simulink model "filtro_ativo"  (R2017a)
settings: Solver=ode3  StartTime=0.0  StopTime=2  MaxStep=Ts  RelTol=1e-3
InitFcn:
  | Ts=1/60/3240;
libraries: powerlib x51, powerlib_meascontrol x3, dsparch4 x2, simulink x1
settings Model: ExtModeTrigMode=oneshot  ExtModeArmWhenConnect=off  ExtModeAutoUpdateStatusClock=off  Creator=patrice  LastModifiedBy=Familia
settings DataIOCC: SaveFormat=Array  SignalLoggingName=sigsOut
settings OptimizationCC: BlockReduction=off  BooleanDataType=off  ExpressionDepthLimit=2147483647  InitFltsAndDblsToZero=on  LifeSpan=inf
settings DebuggingCC: SaveWithParameterizedLinksMsg=none  UnderspecifiedInitializationDetection=Classic  MergeDetectMultiDrivingBlocksExec=none  CheckExecutionContextPreStartOutputMsg=on  CheckExecutionContextRuntimeOutputMsg=on  SignalResolutionControl=TryResolveAllWithWarning  MultiTaskDSMMsg=warning  MultiTaskCondExecSysMsg=none  FcnCallInpInsideContextMsg=warning  StateNameClashWarn=warning  SFUnexpectedBacktrackingDiag=warning  SFNoUnconditionalDefaultTransitionDiag=warning  SFExecutionAtInitializationDiag=none
settings HardwareCC: ProdBitPerPointer=32  ProdBitPerSizeT=32  ProdBitPerPtrDiffT=32  ProdLargestAtomicFloat=None  ProdIntDivRoundTo=Undefined  ProdEndianess=Unspecified  ProdWordSize=32  ProdHWDeviceType=32-bit Generic  TargetUnknown=on
settings ModelReferenceCC: PropagateSignalLabelsOutOfModel=off
settings GRTTargetCC: TargetFcnLib=ansi_tfl_tmw.mat  TargetLangStandard=C89/C90 (ANSI)  GeneratePreprocessorConditionals=Disable all  CombineOutputUpdateFcns=off  GRTInterface=on
settings ConfigComp: CovMetricSettings=dw  CovHtmlReporting=on  CovSaveCumulativeToWorkspaceVar=on  CovSaveSingleToWorkspaceVar=on  CovExternalEMLEnable=off

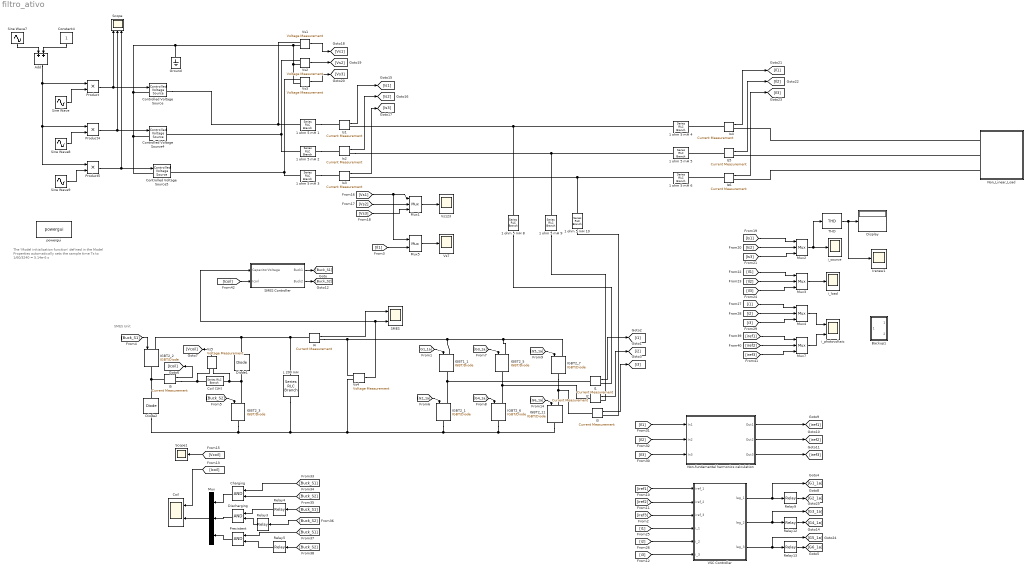
== system filtro_ativo ==
  note: SMES Unit
  note: The 'Model  initialization function' defined in the
      | Model Properties automatically sets the sample time Ts
      | to 1/60/3240 = 5.14e-6 s
  1 ohm 5 mH {1..6} (6 alike) : powerlib/Elements/Series RLC Branch  LConnTagsString=__new0  RConnTagsString=__new0  BranchType=RL  Resistance=0.1  Inductance=0.5e-03  SetiL0=off  InitialCurrent=0  Capacitance=[]  Setx0=off  InitialVoltage=0  Measurements=None
  1 ohm 5 mH 10 : powerlib/Elements/Series RLC Branch  LConnTagsString=__new0  RConnTagsString=__new0  BranchType=RL  Resistance=0.1  Inductance=5e-03  SetiL0=off  InitialCurrent=0  Capacitance=[]  Setx0=off  InitialVoltage=0  Measurements=None
  1 ohm 5 mH 8 : powerlib/Elements/Series RLC Branch  LConnTagsString=__new0  RConnTagsString=__new0  BranchType=RL  Resistance=0.1  Inductance=5e-03  SetiL0=off  InitialCurrent=0  Capacitance=[]  Setx0=off  InitialVoltage=0  Measurements=None
  1 ohm 5 mH 9 : powerlib/Elements/Series RLC Branch  LConnTagsString=__new0  RConnTagsString=__new0  BranchType=RL  Resistance=0.1  Inductance=5e-03  SetiL0=off  InitialCurrent=0  Capacitance=[]  Setx0=off  InitialVoltage=0  Measurements=None
  Add : Sum
  Backup1 : Subsystem
  Charging : Logic  AllPortsSameDT=off
  Coil : Scope  NumInputPorts=2
  "Coil (1H) " : powerlib/Elements/Series RLC Branch  LConnTagsString=__new0  RConnTagsString=__new0  BranchType=L  Resistance=0.1  Inductance=1  SetiL0=on  InitialCurrent=13.2  Capacitance=[]  Setx0=off  InitialVoltage=0  Measurements=None
  Constant4 : Constant
  Controlled Voltage Source : powerlib/Electrical Sources/Controlled Voltage Source  Initialize=on  Source_Type=AC  Amplitude=0  Phase=0  Frequency=0  Measurements=None
  Controlled Voltage Source4 : powerlib/Electrical Sources/Controlled Voltage Source  Initialize=on  Source_Type=AC  Amplitude=0  Phase=0  Frequency=0  Measurements=None
  Controlled Voltage Source5 : powerlib/Electrical Sources/Controlled Voltage Source  Initialize=on  Source_Type=AC  Amplitude=0  Phase=0  Frequency=0  Measurements=None
  Diode1 : powerlib/Power Electronics/Diode  Ron=1e-2  Lon=0  Vf=0.8  IC=0  UseSnubber=off  Rs=inf  Cs=0  Measurements=off
  Diode2 : powerlib/Power Electronics/Diode  Ron=1e-2  Lon=0  Vf=0.8  IC=0  UseSnubber=off  Rs=inf  Cs=0  Measurements=off
  Discharging : Logic  AllPortsSameDT=off
  Display : Display
  Ground : powerlib/Elements/Ground  LConnTagsString=a
  I{1..5} (5 alike) : powerlib/Measurements/Current Measurement  Tag=PoWeRsYsTeMmEaSuReMeNt  PhasorSimulation=off  OutputType=Magnitude  PSBequivalent=0
  IGBT1_1 : powerlib/Power Electronics/IGBT//Diode  Ron=1e-3  Rs=1e5  Cs=inf  Measurements=off
  IGBT2_{1..3,5..7,11} (7 alike) : powerlib/Power Electronics/IGBT//Diode  Ron=1e-3  Rs=1e5  Cs=inf  Measurements=off
  Irenew1 : Scope
  Is{1..6} (6 alike) : powerlib/Measurements/Current Measurement  Tag=PoWeRsYsTeMmEaSuReMeNt  PhasorSimulation=off  OutputType=Magnitude  PSBequivalent=0
  L 200 mH : powerlib/Elements/Series RLC Branch  LConnTagsString=__new0  RConnTagsString=__new0  BranchType=C  Resistance=1.0  Inductance=200e-03  SetiL0=off  InitialCurrent=0  Capacitance=1000e-9  Setx0=on  InitialVoltage=2000  Measurements=None
  Mux{,1..4,7} (6 alike) : Mux  Inputs=3
  Mux5 : Mux  Inputs=2
  Non-fundamental harmonics calculation : Subsystem
  Non_Linear_Load : Subsystem
  Precistent : Logic  AllPortsSameDT=off
  Product : Product
  Product4 : Product
  Product5 : Product
  Relay{3..5,9,12..13} (6 alike) : Relay  OnSwitchValue=0.5  OffSwitchValue=0.5  OnOutputValue=0  OffOutputValue=1
  "SMES " : Scope  NumInputPorts=2
  SMES Controller : Subsystem
  Scope : Scope  NumInputPorts=3
  Scope1 : Scope
  Sine Wave : Sin  Amplitude=230*sqrt(2)  Frequency=100*pi  SampleTime=0
  Sine Wave7 : Sin  Amplitude=0.3  Frequency=2*pi*5  SampleTime=0
  Sine Wave8 : Sin  Amplitude=230*sqrt(2)  Frequency=100*pi  Phase=-2*pi/3  SampleTime=0
  Sine Wave9 : Sin  Amplitude=230*sqrt(2)  Frequency=100*pi  Phase=2*pi/3  SampleTime=0
  THD : powerlib_meascontrol/Measurements/THD  Freq=50  Ts=0
  VSC Controller : Subsystem
  Vs{1..5} (5 alike) : powerlib/Measurements/Voltage Measurement  Tag=PoWeRsYsTeMmEaSuReMeNt  PhasorSimulation=off  OutputType=Magnitude  PSBequivalent=0
  Vs123 : Scope
  Vs7 : Scope
  i_load : Scope
  i_photovoltaic : Scope  NumInputPorts=2
  i_source : Scope
  powergui : powerlib/powergui  SimulationMode=Discrete  SampleTime=Ts  frequency=60  Iterations=50  frequencyindice=0  Pbase=100e6  ErrMax=1e-4  UnitsV=kV  UnitsW=MW  buscounter=0  FunctionMessages=off  echomessages=off  EnableUseOfTLC=off  CurrentSourceSwitches=off  DisableSnubberDevices=off  DisableRonSwitches=off  DisableVfSwitches=off  DisplayEquations=off  SolverType=Tustin  Interpol=off  ExternalGateDelay=off  methode=off  Ts=0  x0status=blocks  SPID=off  SwTol=0  HookPort=off  RestoreLinks=warning  ResistiveCurrentMeasurement=off  Frange=[0:2:500]  Ylog=off  Xlog=on  ShowGrid=off  save=off  variable=ZData  structure=sps1phPWM2_str  ZoomFFT=off  StartTime=0.2  cycles=2  DisplayStyle=2  fundamental=50  FreqAxis=off  MaxFrequency=5000  frequencyindicesteady=1  RmsSteady=1  display=off
  wires:
  [G1_1a] -> IGBT1_1/1
  [G2_1a] -> IGBT2_1/1
  [G3_1a] -> IGBT2_5/1
  [G4_1a] -> IGBT2_6/1
  [G5_1a] -> IGBT2_7/1
  [G6_1a] -> IGBT2_11/1
  I1/1 -> [i1]
  I2/1 -> [i2]
  I3/1 -> [i3]
  Mux1/1 -> Vs123/1
  Is1/1 -> [Is1]
  Is2/1 -> [Is2]
  Is3/1 -> [Is3]
  Vs2/1 -> [Vs2]
  Vs1/1 -> [Vs1]
  Vs3/1 -> [Vs3]
  [Vs1] -> Mux5/1, Mux1/1
  [Vs2] -> Mux1/2
  [Vs3] -> Mux1/3
  Is4/1 -> [Il1]
  Is5/1 -> [Il2]
  Is6/1 -> [Il3]
  [Il1] -> Mux5/2
  Mux5/1 -> Vs7/1
  Mux2/1 -> THD/1, i_source/1
  [Is1] -> Mux2/1
  [Is2] -> Mux2/2
  [Is3] -> Mux2/3
  Mux3/1 -> i_load/1
  [Il2] -> Mux3/2
  [Il3] -> Mux3/3
  Mux4/1 -> i_photovoltaic/1
  [i2] -> Mux4/2
  [i3] -> Mux4/3
  [Il1] -> Mux3/1
  Relay9/1 -> [G2_1a]
  Relay12/1 -> [G4_1a]
  Relay13/1 -> [G6_1a]
  VSC Controller/3(leg_3) -> [G5_1a], Relay13/1
  VSC Controller/1(leg_1) -> Relay9/1, [G1_1a]
  [iref1] -> VSC Controller/1(iref_1)
  [iref3] -> VSC Controller/3(iref_3)
  VSC Controller/2(leg_2) -> Relay12/1, [G3_1a]
  [iref2] -> VSC Controller/2(iref_2)
  [i1] -> VSC Controller/4(i_1)
  [i2] -> VSC Controller/5(i_2)
  [i3] -> VSC Controller/6(i_3)
  THD/1 -> Irenew1/1, Display/1
  Vs4/1 -> "SMES "/2, SMES Controller/1(CapacitorVoltage)
  [i1] -> Mux4/1
  Vs5/1 -> [Vcoil]
  [Buck_S2] -> IGBT2_3/1
  [Buck_S1] -> IGBT2_2/1
  I5/1 -> [Icoil]
  [Icoil] -> Coil/1
  I4/1 -> "SMES "/1
  [Buck_S1] -> Charging/1
  [Buck_S2] -> Charging/2
  [Buck_S1] -> Relay4/1
  [Buck_S2] -> Relay3/1
  Relay4/1 -> Discharging/1
  Relay3/1 -> Discharging/2
  [Buck_S2] -> Relay5/1
  Relay5/1 -> Precistent/2
  [Buck_S1] -> Precistent/1
  Charging/1 -> Mux/1
  Discharging/1 -> Mux/2
  Precistent/1 -> Mux/3
  Mux7/1 -> i_photovoltaic/2
  [iref1] -> Mux7/1
  [iref2] -> Mux7/2
  [iref3] -> Mux7/3
  [Il1] -> Non-fundamental harmonics calculation/1(In1)
  [Il2] -> Non-fundamental harmonics calculation/2(In2)
  [Il3] -> Non-fundamental harmonics calculation/3(In3)
  Non-fundamental harmonics calculation/1(Out1) -> [iref1]
  Non-fundamental harmonics calculation/2(Out2) -> [iref2]
  Non-fundamental harmonics calculation/3(Out3) -> [iref3]
  Constant4/1 -> Add/2
  Sine Wave7/1 -> Add/1
  Sine Wave8/1 -> Product4/2
  Product5/1 -> Controlled Voltage Source5/1, Scope/3
  Sine Wave9/1 -> Product5/2
  Sine Wave/1 -> Product/2
  Product4/1 -> Controlled Voltage Source4/1, Scope/2
  Product/1 -> Controlled Voltage Source/1, Scope/1
  Add/1 -> Product5/1, Product4/1, Product/1
  SMES Controller/1(Buck1) -> [Buck_S1]
  SMES Controller/2(Buck2) -> [Buck_S2]
  [Icoil] -> SMES Controller/2(Icoil)
  [Vcoil] -> Scope1/1
  Mux/1 -> Coil/2
  connections:
  I4/RConn1 -- IGBT1_1/LConn1 -- IGBT2_5/LConn1 -- IGBT2_7/LConn1 -- Vs4/LConn1
  IGBT2_6/LConn1 -- IGBT2_5/RConn1 -- I2/LConn1
  IGBT2_7/RConn1 -- IGBT2_11/LConn1 -- I3/LConn1
  I1/LConn1 -- IGBT1_1/RConn1 -- IGBT2_1/LConn1
  Vs1/LConn1 -- Controlled Voltage Source/RConn1 -- 1 ohm 5 mH 1/LConn1
  1 ohm 5 mH 1/RConn1 -- Is1/LConn1
  1 ohm 5 mH 3/RConn1 -- Is3/LConn1
  1 ohm 5 mH 2/RConn1 -- Is2/LConn1
  1 ohm 5 mH 8/RConn1 -- 1 ohm 5 mH 4/RConn1 -- Is1/RConn1
  Is5/LConn1 -- 1 ohm 5 mH 5/LConn1
  1 ohm 5 mH 6/RConn1 -- Is3/RConn1 -- 1 ohm 5 mH 10/RConn1
  1 ohm 5 mH 8/LConn1 -- I1/RConn1
  1 ohm 5 mH 9/LConn1 -- I2/RConn1
  1 ohm 5 mH 10/LConn1 -- I3/RConn1
  Non_Linear_Load/LConn1 -- Is4/RConn1
  Non_Linear_Load/LConn2 -- Is5/RConn1
  Non_Linear_Load/LConn3 -- Is6/RConn1
  Is4/LConn1 -- 1 ohm 5 mH 4/LConn1
  1 ohm 5 mH 5/RConn1 -- Is2/RConn1 -- 1 ohm 5 mH 9/RConn1
  Is6/LConn1 -- 1 ohm 5 mH 6/LConn1
  I5/LConn1 -- Diode2/RConn1 -- IGBT2_2/RConn1
  IGBT2_3/LConn1 -- Vs5/LConn2 -- "Coil (1H) "/RConn1 -- Diode1/LConn1
  I5/RConn1 -- Vs5/LConn1 -- "Coil (1H) "/LConn1
  L 200 mH/LConn1 -- I4/LConn1 -- Diode1/RConn1 -- IGBT2_2/LConn1
  L 200 mH/RConn1 -- Diode2/LConn1 -- IGBT2_3/RConn1 -- Vs4/LConn2 -- IGBT2_1/RConn1 -- IGBT2_6/RConn1 -- IGBT2_11/RConn1
  Vs2/LConn1 -- 1 ohm 5 mH 2/LConn1 -- Controlled Voltage Source4/RConn1
  Vs3/LConn1 -- 1 ohm 5 mH 3/LConn1 -- Controlled Voltage Source5/RConn1
  Vs3/LConn2 -- Vs2/LConn2 -- Vs1/LConn2 -- Controlled Voltage Source/LConn1 -- Controlled Voltage Source5/LConn1 -- Controlled Voltage Source4/LConn1 -- Ground/LConn1

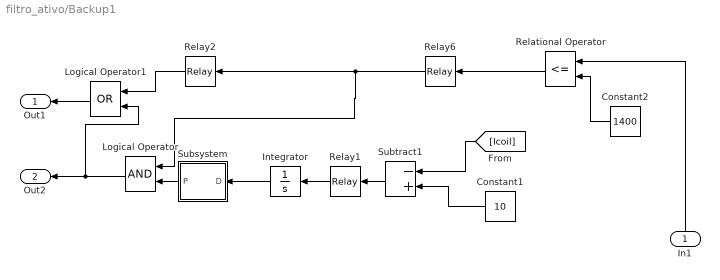
== system filtro_ativo/Backup1 ==
  In1 : Inport
  Constant1 : Constant  Value=10
  Constant2 : Constant  Value=1400
  Integrator : Integrator
  Logical Operator : Logic  AllPortsSameDT=off
  Logical Operator1 : Logic  Operator=OR  AllPortsSameDT=off
  Relational Operator : RelationalOperator  Operator=<=  OutDataTypeStr=boolean  RndMeth=Simplest
  Relay1 : Relay  OnSwitchValue=0.1  OffSwitchValue=-0.1
  Relay2 : Relay  OnSwitchValue=0.5  OffSwitchValue=0.5  OnOutputValue=0  OffOutputValue=1
  Relay6 : Relay  OnSwitchValue=0.1  OffSwitchValue=-0.1
  Subsystem : Subsystem
  Subtract1 : Sum  Inputs=-+
  Out1 : Outport
  Out2 : Outport  Port=2
  wires:
  Relational Operator/1 -> Relay6/1
  Logical Operator1/1 -> Out1/1
  [Icoil] -> Subtract1/1
  Logical Operator/1 -> Out2/1, Logical Operator1/2
  Subtract1/1 -> Relay1/1
  Constant1/1 -> Subtract1/2
  Constant2/1 -> Relational Operator/2
  Relay6/1 -> Logical Operator/1, Relay2/1
  Relay1/1 -> Integrator/1
  Relay2/1 -> Logical Operator1/1
  In1/1 -> Relational Operator/1
  Subsystem/1(P) -> Logical Operator/2
  Integrator/1 -> Subsystem/1(D)

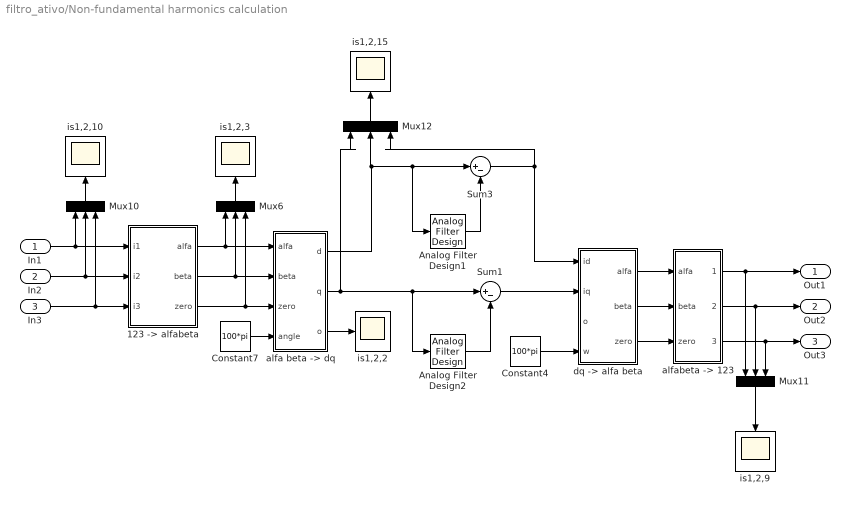
== system filtro_ativo/Non-fundamental harmonics calculation ==
  In1 : Inport
  In2 : Inport  Port=2
  In3 : Inport  Port=3
  "123 -> alfabeta" : Subsystem
  Analog Filter Design1 : dsparch4/Analog Filter Design  method=Butterworth  filttype=Lowpass  N=8  Wlo=2*pi*4  Whi=80  Rp=2  Rs=40
  Analog Filter Design2 : dsparch4/Analog Filter Design  method=Butterworth  filttype=Lowpass  N=8  Wlo=2*pi*4  Whi=80  Rp=2  Rs=40
  Constant4 : Constant  Value=100*pi
  Constant7 : Constant  Value=100*pi
  Mux{6,10..12} (4 alike) : Mux  Inputs=3
  Sum1 : Sum  Inputs=|+-
  Sum3 : Sum  Inputs=|+-
  "alfa beta -> dq" : Subsystem
  "alfabeta -> 123" : Subsystem
  "dq -> alfa beta" : Subsystem
  is1,2,{2..3,9..10,15} (5 alike) : Scope
  Out1 : Outport
  Out2 : Outport  Port=2
  Out3 : Outport  Port=3
  wires:
  "alfa beta -> dq"/3(o) -> is1,2,2/1
  "dq -> alfa beta"/1(alfa) -> "alfabeta -> 123"/1(alfa)
  "dq -> alfa beta"/2(beta) -> "alfabeta -> 123"/2(beta)
  "dq -> alfa beta"/3(zero) -> "alfabeta -> 123"/3(zero)
  Mux10/1 -> is1,2,10/1
  Constant7/1 -> "alfa beta -> dq"/4(angle)
  "123 -> alfabeta"/1(alfa) -> "alfa beta -> dq"/1(alfa), Mux6/1
  "123 -> alfabeta"/2(beta) -> Mux6/2, "alfa beta -> dq"/2(beta)
  "123 -> alfabeta"/3(zero) -> Mux6/3, "alfa beta -> dq"/3(zero)
  Mux12/1 -> is1,2,15/1
  Constant4/1 -> "dq -> alfa beta"/4(w)
  Mux11/1 -> is1,2,9/1
  "alfabeta -> 123"/2(2) -> Out2/1, Mux11/2
  "alfabeta -> 123"/1(1) -> Out1/1, Mux11/1
  "alfabeta -> 123"/3(3) -> Out3/1, Mux11/3
  "alfa beta -> dq"/2(q) -> Mux12/1, Analog Filter Design2/1, Sum1/1
  In3/1 -> "123 -> alfabeta"/3(i3), Mux10/3
  Mux6/1 -> is1,2,3/1
  Analog Filter Design1/1 -> Sum3/2
  Analog Filter Design2/1 -> Sum1/2
  In1/1 -> "123 -> alfabeta"/1(i1), Mux10/1
  In2/1 -> "123 -> alfabeta"/2(i2), Mux10/2
  "alfa beta -> dq"/1(d) -> Sum3/1, Analog Filter Design1/1, Mux12/2
  Sum1/1 -> "dq -> alfa beta"/2(iq)
  Sum3/1 -> Mux12/3, "dq -> alfa beta"/1(id)

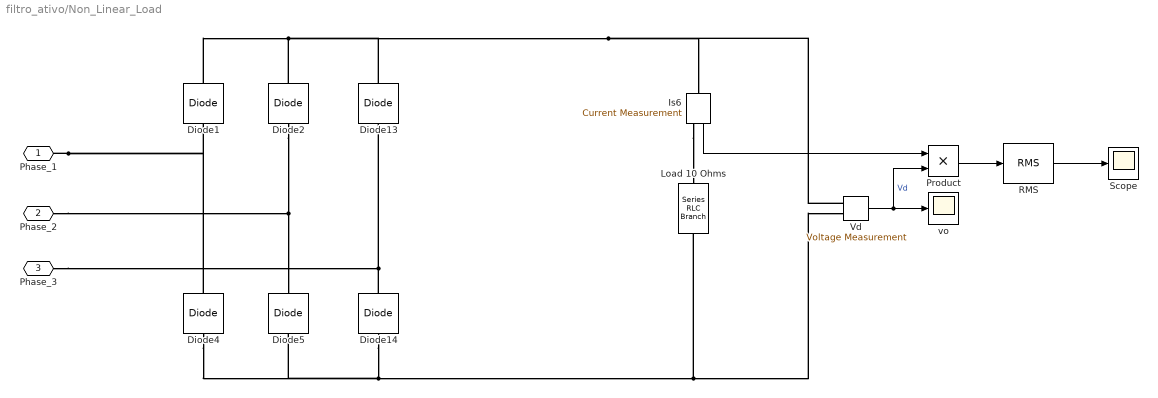
== system filtro_ativo/Non_Linear_Load ==
  Diode{1..2,4..5,13..14} (6 alike) : powerlib/Power Electronics/Diode  Ron=1e-2  Lon=0  Vf=0.8  IC=0  UseSnubber=off  Rs=1000  Cs=0.1e-6  Measurements=off
  Is6 : powerlib/Measurements/Current Measurement  Tag=PoWeRsYsTeMmEaSuReMeNt  PhasorSimulation=off  OutputType=Magnitude  PSBequivalent=0
  Load 10 Ohms : powerlib/Elements/Series RLC Branch  LConnTagsString=__new0  RConnTagsString=__new0  BranchType=R  Resistance=60  Inductance=1.0  SetiL0=off  InitialCurrent=0  Capacitance=1.0  Setx0=off  InitialVoltage=0  Measurements=None
  Product : Product
  RMS : powerlib_meascontrol/Measurements/RMS  TrueRMS=on  Freq=60  RMSInit=120  Ts=0
  Scope : Scope
  Vd : powerlib/Measurements/Voltage Measurement  Tag=PoWeRsYsTeMmEaSuReMeNt  PhasorSimulation=off  OutputType=Magnitude  PSBequivalent=0
  vo : Scope
  Phase_1 : PMIOPort  Port=1  Side=Left
  Phase_2 : PMIOPort  Port=2  Side=Left
  Phase_3 : PMIOPort  Port=3  Side=Left
  wires:
  Vd/1 -> Product/2, vo/1  "Vd"
  Is6/1 -> Product/1
  Product/1 -> RMS/1
  RMS/1 -> Scope/1
  connections:
  Phase_1/RConn1 -- Diode4/RConn1 -- Diode1/LConn1
  Diode1/RConn1 -- Diode13/RConn1 -- Is6/LConn1 -- Vd/LConn1 -- Diode2/RConn1
  Diode2/LConn1 -- Phase_2/RConn1 -- Diode5/RConn1
  Diode14/RConn1 -- Phase_3/RConn1 -- Diode13/LConn1
  Diode14/LConn1 -- Diode4/LConn1 -- Diode5/LConn1 -- Vd/LConn2 -- Load 10 Ohms/RConn1
  Is6/RConn1 -- Load 10 Ohms/LConn1

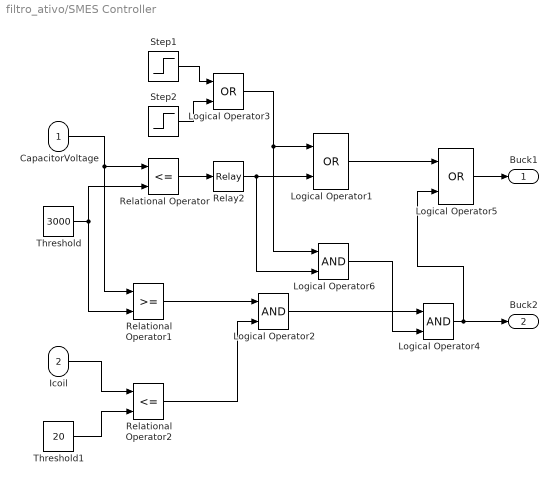
== system filtro_ativo/SMES Controller ==
  CapacitorVoltage : Inport
  Icoil : Inport  Port=2
  Logical Operator1 : Logic  Operator=OR  AllPortsSameDT=off
  Logical Operator2 : Logic  AllPortsSameDT=off
  Logical Operator3 : Logic  Operator=OR  AllPortsSameDT=off
  Logical Operator4 : Logic  AllPortsSameDT=off
  Logical Operator5 : Logic  Operator=OR  AllPortsSameDT=off
  Logical Operator6 : Logic  AllPortsSameDT=off
  Relational Operator : RelationalOperator  Operator=<=  OutDataTypeStr=boolean  RndMeth=Simplest
  Relational Operator1 : RelationalOperator  OutDataTypeStr=boolean  RndMeth=Simplest
  Relational Operator2 : RelationalOperator  Operator=<=  OutDataTypeStr=boolean  RndMeth=Simplest
  Relay2 : Relay  OnSwitchValue=0.5  OffSwitchValue=0.5  OnOutputValue=0  OffOutputValue=1
  Step1 : Step  Time=0.52  Before=1  After=0  SampleTime=0
  Step2 : Step  Time=0.98  SampleTime=0
  Threshold : Constant  Value=3000
  Threshold1 : Constant  Value=20
  Buck1 : Outport
  Buck2 : Outport  Port=2
  wires:
  CapacitorVoltage/1 -> Relational Operator1/1, Relational Operator/1
  Step2/1 -> Logical Operator3/2
  Logical Operator1/1 -> Logical Operator5/1
  Threshold/1 -> Relational Operator1/2, Relational Operator/2
  Relational Operator/1 -> Relay2/1
  Step1/1 -> Logical Operator3/1
  Relay2/1 -> Logical Operator1/2, Logical Operator6/2
  Logical Operator3/1 -> Logical Operator6/1, Logical Operator1/1
  Relational Operator1/1 -> Logical Operator2/1
  Icoil/1 -> Relational Operator2/1
  Threshold1/1 -> Relational Operator2/2
  Logical Operator2/1 -> Logical Operator4/1
  Logical Operator4/1 -> Logical Operator5/2, Buck2/1
  Relational Operator2/1 -> Logical Operator2/2
  Logical Operator5/1 -> Buck1/1
  Logical Operator6/1 -> Logical Operator4/2

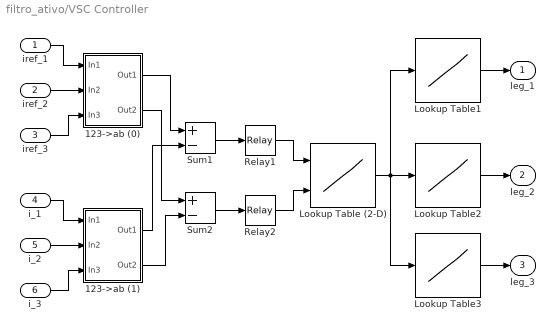
== system filtro_ativo/VSC Controller ==
  iref_1 : Inport
  iref_2 : Inport  Port=2
  iref_3 : Inport  Port=3
  i_1 : Inport  Port=4
  i_2 : Inport  Port=5
  i_3 : Inport  Port=6
  123->ab (0) : Subsystem
  123->ab (1) : Subsystem
  Lookup Table (2-D) : Lookup2D  RowIndex=[0:1]  ColumnIndex=[0:1]  Table=[5 3;6 2]
  Lookup Table1 : Lookup  InputValues=[0:6]  Table=[0 1 1 0 0 0 1]
  Lookup Table2 : Lookup  InputValues=[0:6]  Table=[0 0 1 1 1 0 0]
  Lookup Table3 : Lookup  InputValues=[0:6]  Table=[0 0 0 0 1 1 1]
  Relay1 : Relay  OnSwitchValue=0.01  OffSwitchValue=-0.01
  Relay2 : Relay  OnSwitchValue=0.01  OffSwitchValue=-0.01
  Sum1 : Sum  Inputs=+-  SaturateOnIntegerOverflow=on  InputSameDT=on  OutDataTypeStr=Inherit: Same as first input
  Sum2 : Sum  Inputs=+-  SaturateOnIntegerOverflow=on  InputSameDT=on  OutDataTypeStr=Inherit: Same as first input
  leg_1 : Outport
  leg_2 : Outport  Port=2
  leg_3 : Outport  Port=3
  wires:
  Relay2/1 -> Lookup Table (2-D)/2
  123->ab (1)/2(Out2) -> Sum2/2
  Relay1/1 -> Lookup Table (2-D)/1
  Sum2/1 -> Relay2/1
  Sum1/1 -> Relay1/1
  123->ab (0)/1(Out1) -> Sum1/1
  i_3/1 -> 123->ab (1)/3(In3)
  i_2/1 -> 123->ab (1)/2(In2)
  Lookup Table2/1 -> leg_2/1
  Lookup Table3/1 -> leg_3/1
  iref_2/1 -> 123->ab (0)/2(In2)
  Lookup Table1/1 -> leg_1/1
  123->ab (1)/1(Out1) -> Sum1/2
  iref_1/1 -> 123->ab (0)/1(In1)
  iref_3/1 -> 123->ab (0)/3(In3)
  i_1/1 -> 123->ab (1)/1(In1)
  123->ab (0)/2(Out2) -> Sum2/1
  Lookup Table (2-D)/1 -> Lookup Table1/1, Lookup Table2/1, Lookup Table3/1

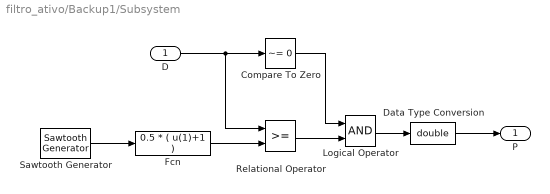
== system filtro_ativo/Backup1/Subsystem ==
  D : Inport  SampleTime=Ts
  Compare To Zero : simulink/Logic and Bit Operations/Compare To Zero  relop=~=  OutDataTypeStr=boolean
  Data Type Conversion : DataTypeConversion  OutDataTypeStr=double
  Fcn : Fcn  Expr=0.5 * ( u(1)+1 )
  Logical Operator : Logic  AllPortsSameDT=off  OutDataTypeStr=boolean
  Relational Operator : RelationalOperator  OutDataTypeStr=boolean  RndMeth=Nearest
  Sawtooth Generator : powerlib_meascontrol/Pulse & Signal Generators/Sawtooth Generator  Freq=500  Phase=0  Ts=Ts
      settings: SourceProductName=Simscape Power Systems
  P : Outport
  wires:
  Logical Operator/1 -> Data Type Conversion/1
  Compare To Zero/1 -> Logical Operator/1
  Data Type Conversion/1 -> P/1
  Sawtooth Generator/1 -> Fcn/1
  Fcn/1 -> Relational Operator/2
  D/1 -> Compare To Zero/1, Relational Operator/1
  Relational Operator/1 -> Logical Operator/2

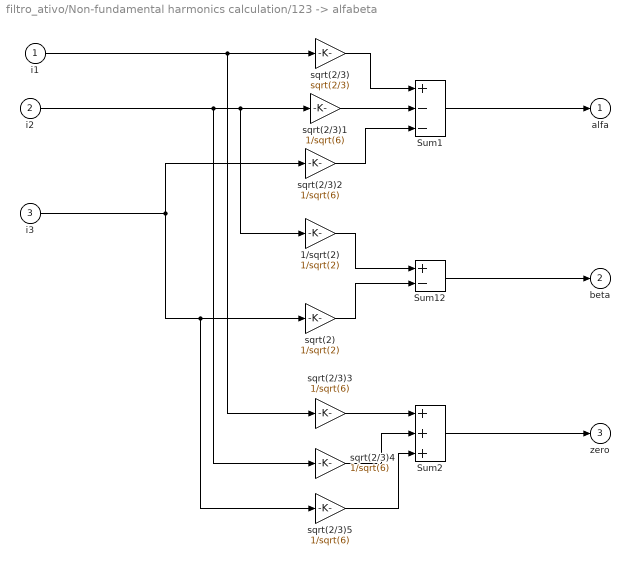
== system filtro_ativo/Non-fundamental harmonics calculation/123 -> alfabeta ==
  i1 : Inport
  i2 : Inport  Port=2
  i3 : Inport  Port=3
  1/sqrt(2) : Gain  Gain=1/sqrt(2)  SaturateOnIntegerOverflow=on  OutDataTypeStr=Inherit: Same as input  ParamDataTypeStr=Inherit: Same as input
  Sum1 : Sum  Inputs=+--  SaturateOnIntegerOverflow=on  InputSameDT=on  OutDataTypeStr=Inherit: Same as first input
  Sum12 : Sum  Inputs=+-  SaturateOnIntegerOverflow=on  InputSameDT=on  OutDataTypeStr=Inherit: Same as first input
  Sum2 : Sum  Inputs=+++  SaturateOnIntegerOverflow=on  InputSameDT=on  OutDataTypeStr=Inherit: Same as first input
  sqrt(2) : Gain  Gain=1/sqrt(2)  SaturateOnIntegerOverflow=on  OutDataTypeStr=Inherit: Same as input  ParamDataTypeStr=Inherit: Same as input
  sqrt(2/3) : Gain  Gain=sqrt(2/3)  SaturateOnIntegerOverflow=on  OutDataTypeStr=Inherit: Same as input  ParamDataTypeStr=Inherit: Same as input
  sqrt(2/3){1..5} (5 alike) : Gain  Gain=1/sqrt(6)  SaturateOnIntegerOverflow=on  OutDataTypeStr=Inherit: Same as input  ParamDataTypeStr=Inherit: Same as input
  alfa : Outport  InitialOutput=0
  beta : Outport  Port=2  InitialOutput=0
  zero : Outport  Port=3  InitialOutput=0
  wires:
  i1/1 -> sqrt(2/3)3/1, sqrt(2/3)/1
  1/sqrt(2)/1 -> Sum12/1
  sqrt(2)/1 -> Sum12/2
  Sum12/1 -> beta/1
  i2/1 -> sqrt(2/3)4/1, sqrt(2/3)1/1, 1/sqrt(2)/1
  i3/1 -> sqrt(2/3)2/1, sqrt(2/3)5/1, sqrt(2)/1
  sqrt(2/3)2/1 -> Sum1/3
  sqrt(2/3)1/1 -> Sum1/2
  sqrt(2/3)/1 -> Sum1/1
  Sum1/1 -> alfa/1
  sqrt(2/3)3/1 -> Sum2/1
  sqrt(2/3)4/1 -> Sum2/2
  sqrt(2/3)5/1 -> Sum2/3
  Sum2/1 -> zero/1

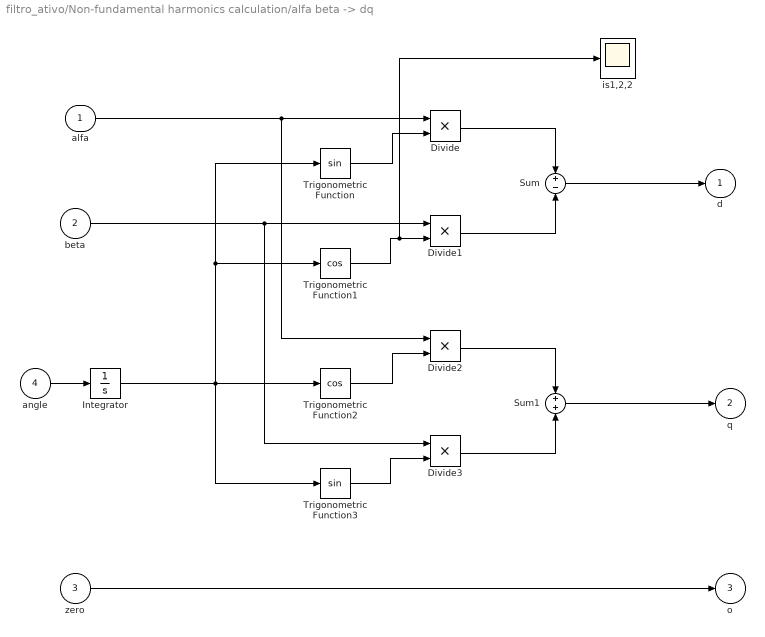
== system filtro_ativo/Non-fundamental harmonics calculation/alfa beta -> dq ==
  alfa : Inport
  beta : Inport  Port=2
  zero : Inport  Port=3
  angle : Inport  Port=4
  Divide{,1..3} (4 alike) : Product  Inputs=**
  Integrator : Integrator
  Sum : Sum  Inputs=+-
  Sum1 : Sum
  Trigonometric Function : Trigonometry
  Trigonometric Function1 : Trigonometry  Operator=cos
  Trigonometric Function2 : Trigonometry  Operator=cos
  Trigonometric Function3 : Trigonometry
  is1,2,2 : Scope
  d : Outport  InitialOutput=0
  q : Outport  Port=2  InitialOutput=0
  o : Outport  Port=3  InitialOutput=0
  wires:
  angle/1 -> Integrator/1
  alfa/1 -> Divide2/1, Divide/1
  Trigonometric Function/1 -> Divide/2
  beta/1 -> Divide3/1, Divide1/1
  Trigonometric Function1/1 -> is1,2,2/1, Divide1/2
  Divide/1 -> Sum/1
  Divide1/1 -> Sum/2
  Trigonometric Function2/1 -> Divide2/2
  Trigonometric Function3/1 -> Divide3/2
  Divide2/1 -> Sum1/1
  Divide3/1 -> Sum1/2
  Sum/1 -> d/1
  Sum1/1 -> q/1
  zero/1 -> o/1
  Integrator/1 -> Trigonometric Function3/1, Trigonometric Function1/1, Trigonometric Function/1, Trigonometric Function2/1

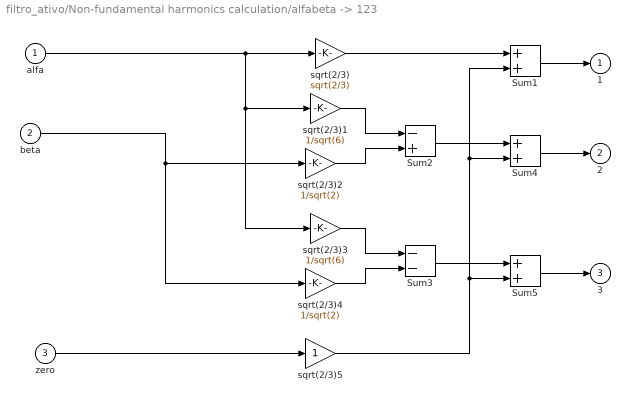
== system filtro_ativo/Non-fundamental harmonics calculation/alfabeta -> 123 ==
  alfa : Inport
  beta : Inport  Port=2
  zero : Inport  Port=3
  Sum1 : Sum  SaturateOnIntegerOverflow=on  InputSameDT=on  OutDataTypeStr=Inherit: Same as first input
  Sum2 : Sum  Inputs=-+  SaturateOnIntegerOverflow=on  InputSameDT=on  OutDataTypeStr=Inherit: Same as first input
  Sum3 : Sum  Inputs=--  SaturateOnIntegerOverflow=on  InputSameDT=on  OutDataTypeStr=Inherit: Same as first input
  Sum4 : Sum  SaturateOnIntegerOverflow=on  InputSameDT=on  OutDataTypeStr=Inherit: Same as first input
  Sum5 : Sum  SaturateOnIntegerOverflow=on  InputSameDT=on  OutDataTypeStr=Inherit: Same as first input
  sqrt(2/3) : Gain  Gain=sqrt(2/3)  SaturateOnIntegerOverflow=on  OutDataTypeStr=Inherit: Same as input  ParamDataTypeStr=Inherit: Same as input
  sqrt(2/3)1 : Gain  Gain=1/sqrt(6)  SaturateOnIntegerOverflow=on  OutDataTypeStr=Inherit: Same as input  ParamDataTypeStr=Inherit: Same as input
  sqrt(2/3)2 : Gain  Gain=1/sqrt(2)  SaturateOnIntegerOverflow=on  OutDataTypeStr=Inherit: Same as input  ParamDataTypeStr=Inherit: Same as input
  sqrt(2/3)3 : Gain  Gain=1/sqrt(6)  SaturateOnIntegerOverflow=on  OutDataTypeStr=Inherit: Same as input  ParamDataTypeStr=Inherit: Same as input
  sqrt(2/3)4 : Gain  Gain=1/sqrt(2)  SaturateOnIntegerOverflow=on  OutDataTypeStr=Inherit: Same as input  ParamDataTypeStr=Inherit: Same as input
  sqrt(2/3)5 : Gain  SaturateOnIntegerOverflow=on  OutDataTypeStr=Inherit: Same as input  ParamDataTypeStr=Inherit: Same as input
  1 : Outport  InitialOutput=0
  2 : Outport  Port=2  InitialOutput=0
  3 : Outport  Port=3  InitialOutput=0
  wires:
  sqrt(2/3)5/1 -> Sum1/2, Sum4/2, Sum5/2
  Sum5/1 -> 3/1
  Sum3/1 -> Sum5/1
  Sum4/1 -> 2/1
  Sum2/1 -> Sum4/1
  zero/1 -> sqrt(2/3)5/1
  Sum1/1 -> 1/1
  sqrt(2/3)/1 -> Sum1/1
  alfa/1 -> sqrt(2/3)/1, sqrt(2/3)1/1, sqrt(2/3)3/1
  beta/1 -> sqrt(2/3)2/1, sqrt(2/3)4/1
  sqrt(2/3)2/1 -> Sum2/2
  sqrt(2/3)1/1 -> Sum2/1
  sqrt(2/3)4/1 -> Sum3/2
  sqrt(2/3)3/1 -> Sum3/1

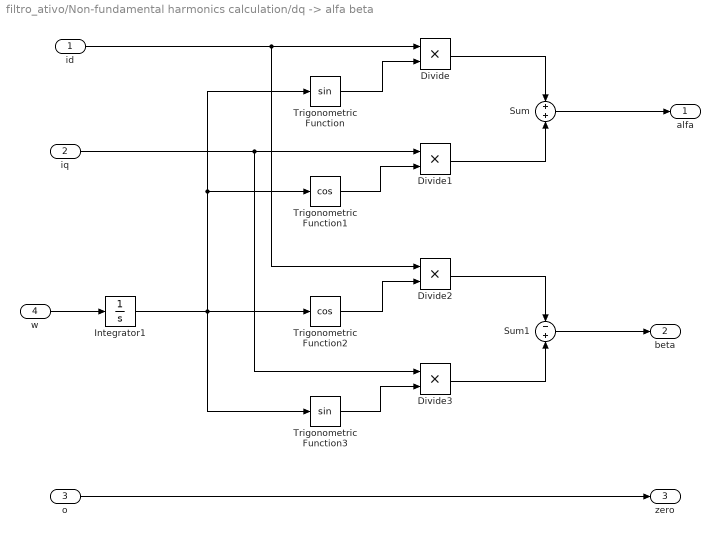
== system filtro_ativo/Non-fundamental harmonics calculation/dq -> alfa beta ==
  id : Inport
  iq : Inport  Port=2
  o : Inport  Port=3
  w : Inport  Port=4
  Divide{,1..3} (4 alike) : Product  Inputs=**
  Integrator1 : Integrator
  Sum : Sum
  Sum1 : Sum  Inputs=-+
  Trigonometric Function : Trigonometry
  Trigonometric Function1 : Trigonometry  Operator=cos
  Trigonometric Function2 : Trigonometry  Operator=cos
  Trigonometric Function3 : Trigonometry
  alfa : Outport
  beta : Outport  Port=2
  zero : Outport  Port=3
  wires:
  o/1 -> zero/1
  Sum1/1 -> beta/1
  Sum/1 -> alfa/1
  Divide3/1 -> Sum1/2
  Divide2/1 -> Sum1/1
  Trigonometric Function3/1 -> Divide3/2
  Trigonometric Function2/1 -> Divide2/2
  Divide1/1 -> Sum/2
  Divide/1 -> Sum/1
  Trigonometric Function1/1 -> Divide1/2
  iq/1 -> Divide1/1, Divide3/1
  Trigonometric Function/1 -> Divide/2
  id/1 -> Divide/1, Divide2/1
  w/1 -> Integrator1/1
  Integrator1/1 -> Trigonometric Function3/1, Trigonometric Function1/1, Trigonometric Function/1, Trigonometric Function2/1

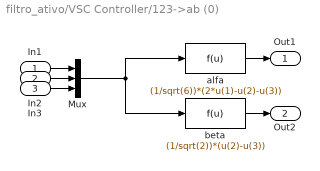
== system filtro_ativo/VSC Controller/123->ab (0) ==
  In1 : Inport
  In2 : Inport  Port=2
  In3 : Inport  Port=3
  Mux : Mux  Inputs=3
  alfa : Fcn  Expr=(1/sqrt(6))*(2*u(1)-u(2)-u(3))
  beta : Fcn  Expr=(1/sqrt(2))*(u(2)-u(3))
  Out1 : Outport
  Out2 : Outport  Port=2
  wires:
  Mux/1 -> beta/1, alfa/1
  alfa/1 -> Out1/1
  In1/1 -> Mux/1
  In2/1 -> Mux/2
  In3/1 -> Mux/3
  beta/1 -> Out2/1

== system filtro_ativo/VSC Controller/123->ab (1) ==
  In1 : Inport
  In2 : Inport  Port=2
  In3 : Inport  Port=3
  Mux : Mux  Inputs=3
  alfa : Fcn  Expr=(1/sqrt(6))*(2*u(1)-u(2)-u(3))
  beta : Fcn  Expr=(1/sqrt(2))*(u(2)-u(3))
  Out1 : Outport
  Out2 : Outport  Port=2
  wires:
  beta/1 -> Out2/1
  In3/1 -> Mux/3
  In2/1 -> Mux/2
  In1/1 -> Mux/1
  alfa/1 -> Out1/1
  Mux/1 -> alfa/1, beta/1
